simulink model "CruiseControl"  (R2024a)
settings: Solver=ode3  StartTime=0.0  StopTime=32  FixedStep=0.01  RelTol=1e-3
undefined symbols (not defined in the file): magnitude
libraries: simulink x8, SignalEditorBlockLib x1, slpidlib x1
settings Model: Creator=bnoo3  LastModifiedBy=oyj92
settings DataIOCC: SaveFormat=Array
settings ModelReferenceCC: EnableRefExpFcnMdlSchedulingChecks=on

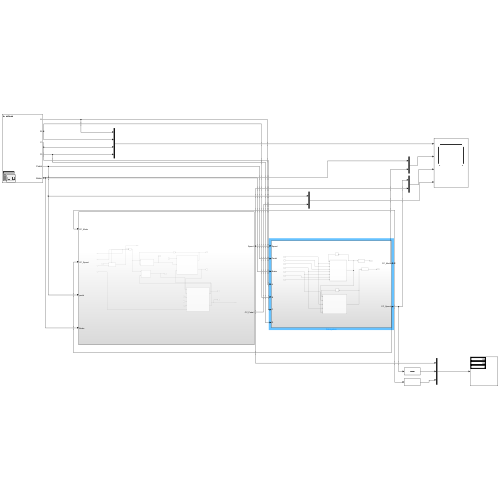
[thumbnail: Simulink's stored preview of the top-level diagram]
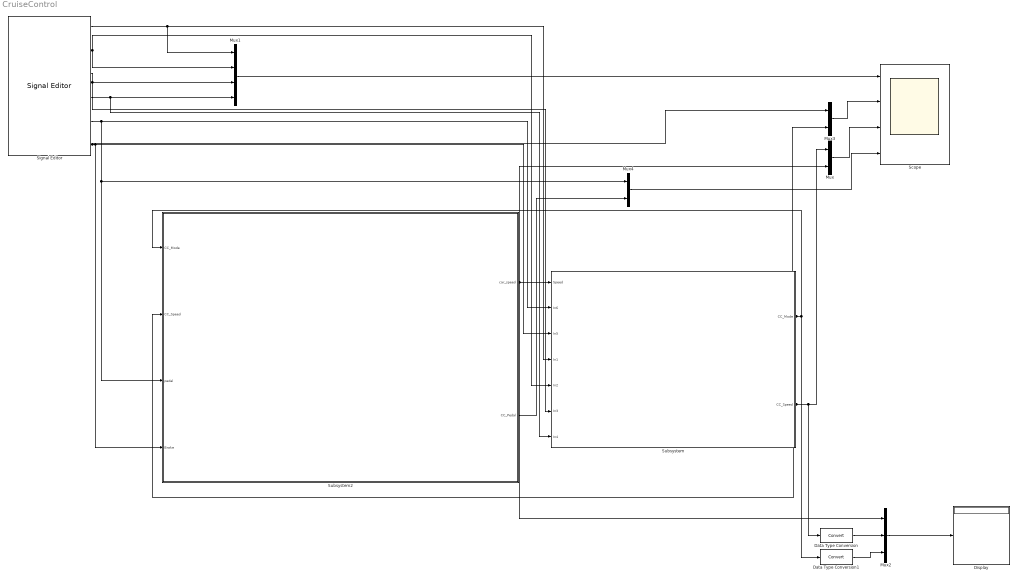
== system CruiseControl ==
  Data Type Conversion : DataTypeConversion  SaturateOnIntegerOverflow=off  RndMeth=Floor
  Data Type Conversion1 : DataTypeConversion  SaturateOnIntegerOverflow=off  RndMeth=Floor
  Display : Display
  Mux : Mux  Inputs=2
  Mux1 : Mux
  Mux2 : Mux  Inputs=3
  Mux3 : Mux  Inputs=2
  Mux4 : Mux  Inputs=2
  Scope : Scope  NumInputPorts=4
  Signal Editor : SignalEditorBlockLib/Signal Editor  FileName=C:\Users\oyj92\OneDrive\바탕 화면\OneDrive\대학교\2024-2\전장시\Ch8_CruiseControl\ref\Scenario_Result\Scenario2.mat  ActiveScenario=Scenario2  ActiveSignal=Brake  IsBus=off  OutputBusObjectStr=Bus: BusObject  SampleTime=0  Interpolate=off  ZeroCross=off  OutputAfterFinalValue=Setting to zero  Unit=inherit  PreserveSignalName=on  ApplySigPropsToAllScenarios=on  ApplySigPropsToAllSignals=off
  Subsystem : Subsystem
  Subsystem2 : Subsystem
  wires:
  Signal Editor/2 -> Mux1/2, Subsystem/5(In2)
  Signal Editor/4 -> Subsystem/7(In4), Mux1/4
  Signal Editor/6 -> Subsystem2/4(Brake), Subsystem/3(In5), Mux3/1
  Signal Editor/1 -> Subsystem/4(In1), Mux1/1
  Signal Editor/3 -> Mux1/3, Subsystem/6(In3)
  Signal Editor/5 -> Subsystem2/3(pedal), Mux4/1, Subsystem/2(In6)
  Mux/1 -> Scope/3
  Mux1/1 -> Scope/1
  Subsystem2/1(car_speed) -> Mux/2, Mux2/1, Subsystem/1(Speed)
  Subsystem2/2(CC_Pedal) -> Mux4/2
  Mux4/1 -> Scope/4
  Subsystem/1(CC_Mode) -> Mux3/2, Subsystem2/1(CC_Mode), Data Type Conversion1/1
  Subsystem/2(CC_Speed) -> Subsystem2/2(CC_Speed), Mux/1, Data Type Conversion/1
  Mux3/1 -> Scope/2
  Data Type Conversion1/1 -> Mux2/3
  Data Type Conversion/1 -> Mux2/2
  Mux2/1 -> Display/1

== system CruiseControl/Subsystem ==
  Speed : Inport
  In6 : Inport  Port=2
  In5 : Inport  Port=3
  In1 : Inport  Port=4
  In2 : Inport  Port=5
  In3 : Inport  Port=6
  In4 : Inport  Port=7
  CC ON/OFF : Subsystem
  CC SPEED Calculator : Subsystem
  Data Type Conversion : DataTypeConversion  SaturateOnIntegerOverflow=off  RndMeth=Floor
  Data Type Conversion1 : DataTypeConversion  SaturateOnIntegerOverflow=off  RndMeth=Floor
  Unit Delay : UnitDelay  SampleTime=0.01  HasFrameUpgradeWarning=on
  Unit Delay1 : UnitDelay  SampleTime=0.01  HasFrameUpgradeWarning=on
  CC_Mode : Outport
  CC_Speed : Outport  Port=2  OutMin=0  OutMax=255  OutDataTypeStr=int16
  wires:
  CC ON/OFF/1(CC_Mode) -> CC SPEED Calculator/2(Speed), Unit Delay/1, Data Type Conversion/1
  In1/1 -> CC SPEED Calculator/4(A), CC ON/OFF/5(In3)  "A"
  In2/1 -> CC SPEED Calculator/5(B), CC ON/OFF/6(In4)  "B"
  In3/1 -> CC ON/OFF/7(In5)  "C"
  In5/1 -> CC ON/OFF/4(Brake)  "Brake"
  Unit Delay/1 -> CC ON/OFF/1(In1)
  In4/1 -> CC ON/OFF/8(In6)  "D"
  Speed/1 -> CC SPEED Calculator/3(In2), CC ON/OFF/2(Speed)  "Speed"
  In6/1 -> CC ON/OFF/3(Pedal)  "Pedal"
  CC SPEED Calculator/1(CC_speed) -> Unit Delay1/1, Data Type Conversion1/1
  Unit Delay1/1 -> CC SPEED Calculator/1(In1)
  Data Type Conversion/1 -> CC_Mode/1  "CC_Mode"
  Data Type Conversion1/1 -> CC_Speed/1  "CC_Speed"

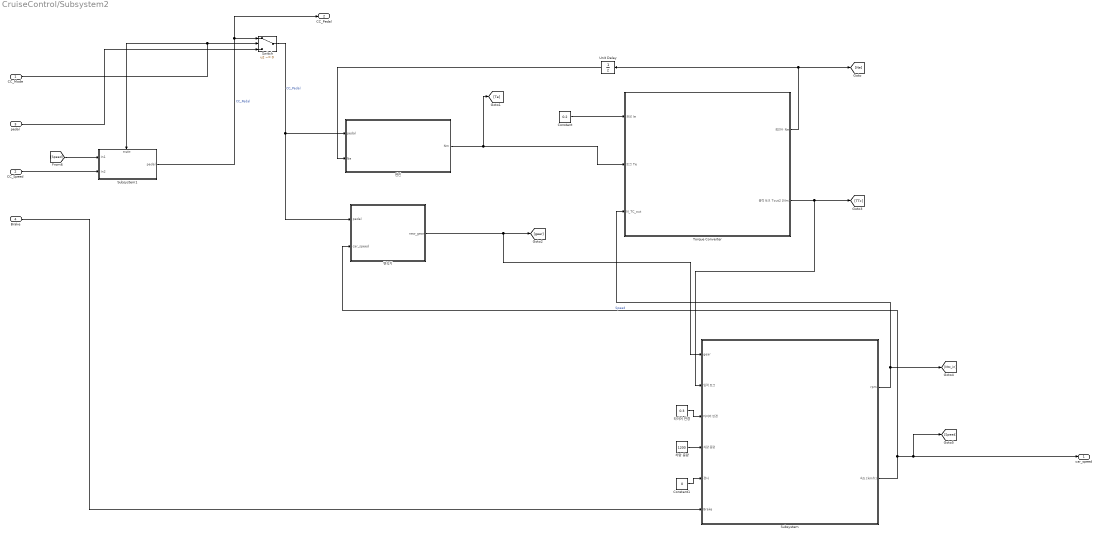
== system CruiseControl/Subsystem2 ==
  CC_Mode : Inport
  CC_Speed : Inport  Port=2
  pedal : Inport  Port=3
  Brake : Inport  Port=4
  Constant : Constant  Value=0.2
  Constant1 : Constant  Value=0
  Subsystem : Subsystem
  Subsystem1 : Subsystem
  Switch : Switch  Criteria=u2 ~= 0  SaturateOnIntegerOverflow=off  InputSameDT=off
  Torque Converter : Subsystem
  Unit Delay : UnitDelay  SampleTime=-1  HasFrameUpgradeWarning=on
  변속기 : Subsystem
  엔진 : Subsystem
  차량 중량 : Constant  Value=1200
  타이어 반경 : Constant  Value=0.3
  car_speed : Outport
  CC_Pedal : Outport  Port=2
  wires:
  Switch/1 -> 엔진/1(pedal), 변속기/1(pedal)  "CC_Pedal"
  CC_Mode/1 -> Subsystem1/Enable, Switch/2
  Unit Delay/1 -> 엔진/2(Ne)
  Subsystem/2(속도 [km/h]) -> 변속기/2(car_speed), car_speed/1, [Speed]  "Speed"
  타이어 반경/1 -> Subsystem/3(타이어 반경)
  CC_Speed/1 -> Subsystem1/2(In2)
  엔진/1(Nm) -> [Te], Torque Converter/2(토크 Te)
  pedal/1 -> Switch/3
  변속기/1(new_gear) -> [gear], Subsystem/1(gear)
  Constant1/1 -> Subsystem/5(경사)
  Torque Converter/2(출력 토크 Tout2 [Nm]) -> [TTc], Subsystem/2(입력 토크)
  Subsystem1/1(pedal) -> CC_Pedal/1, Switch/1  "CC_Pedal"
  Brake/1 -> Subsystem/6(Brake)
  Constant/1 -> Torque Converter/1(관성 Ie)
  Subsystem/1(rpm) -> Torque Converter/3(N_TC_out), [Ntc_in]
  Torque Converter/1(회전수 Ne) -> Unit Delay/1, [Ne]
  [Speed] -> Subsystem1/1(In1)
  차량 중량/1 -> Subsystem/4(차량 중량)

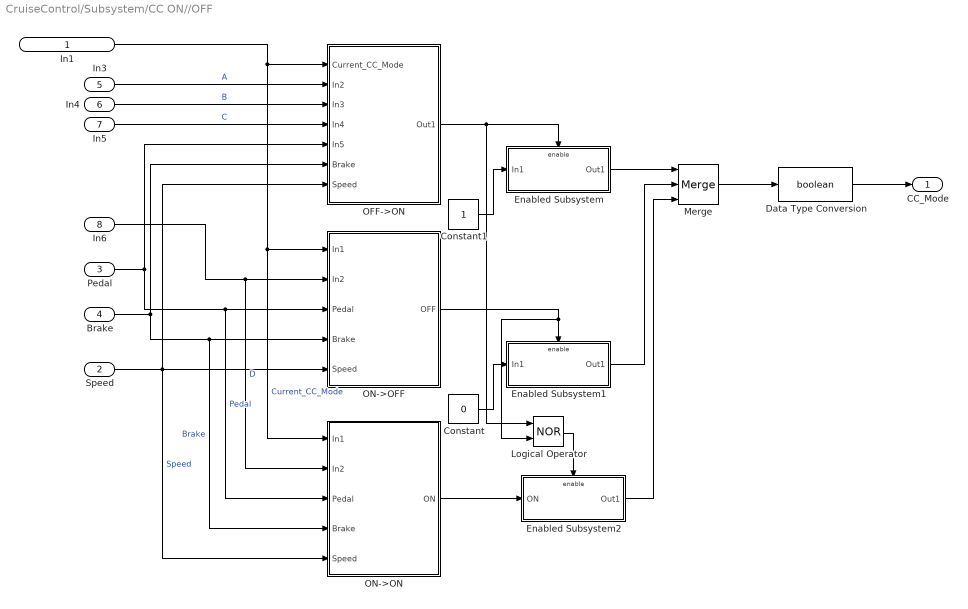
== system CruiseControl/Subsystem/CC ON//OFF ==
  In1 : Inport
  Speed : Inport  Port=2
  Pedal : Inport  Port=3
  Brake : Inport  Port=4
  In3 : Inport  Port=5
  In4 : Inport  Port=6
  In5 : Inport  Port=7
  In6 : Inport  Port=8
  Constant : Constant  Value=0
  Constant1 : Constant
  Data Type Conversion : DataTypeConversion  OutDataTypeStr=boolean  SaturateOnIntegerOverflow=off  RndMeth=Floor
  Enabled Subsystem : Subsystem  TreatAsAtomicUnit=on
  Enabled Subsystem1 : Subsystem  TreatAsAtomicUnit=on
  Enabled Subsystem2 : Subsystem  TreatAsAtomicUnit=on
  Logical Operator : Logic  Operator=NOR  AllPortsSameDT=off  OutDataTypeStr=boolean
  Merge : Merge  Inputs=3
  OFF->ON : Subsystem
  ON->OFF : Subsystem
  ON->ON : Subsystem
  CC_Mode : Outport
  wires:
  Data Type Conversion/1 -> CC_Mode/1
  ON->ON/1(ON) -> Enabled Subsystem2/1(ON)
  Enabled Subsystem2/1(Out1) -> Merge/3
  Speed/1 -> OFF->ON/7(Speed), ON->ON/5(Speed), ON->OFF/5(Speed)  "Speed"
  Enabled Subsystem/1(Out1) -> Merge/1
  In1/1 -> ON->ON/1(In1), ON->OFF/1(In1), OFF->ON/1(Current_CC_Mode)  "Current_CC_Mode"
  Enabled Subsystem1/1(Out1) -> Merge/2
  Merge/1 -> Data Type Conversion/1
  In5/1 -> OFF->ON/4(In4)  "C"
  In3/1 -> OFF->ON/2(In2)  "A"
  OFF->ON/1(Out1) -> Enabled Subsystem/Enable, Logical Operator/1
  Pedal/1 -> ON->ON/3(Pedal), ON->OFF/3(Pedal), OFF->ON/5(In5)  "Pedal"
  In6/1 -> ON->ON/2(In2), ON->OFF/2(In2)  "D"
  ON->OFF/1(OFF) -> Logical Operator/2, Enabled Subsystem1/Enable
  Constant/1 -> Enabled Subsystem1/1(In1)
  Brake/1 -> ON->ON/4(Brake), ON->OFF/4(Brake), OFF->ON/6(Brake)  "Brake"
  Constant1/1 -> Enabled Subsystem/1(In1)
  In4/1 -> OFF->ON/3(In3)  "B"
  Logical Operator/1 -> Enabled Subsystem2/Enable

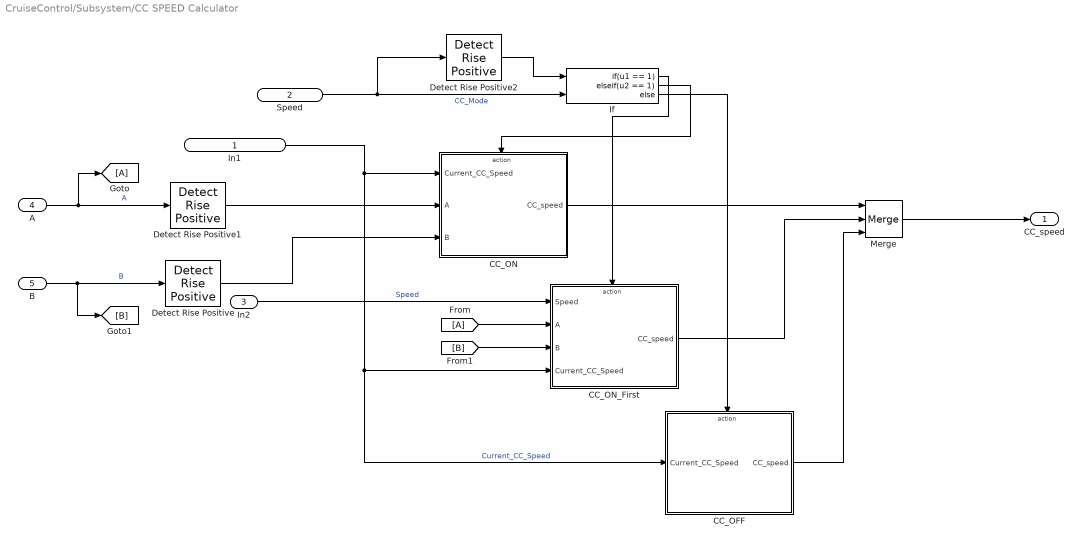
== system CruiseControl/Subsystem/CC SPEED Calculator ==
  In1 : Inport
  Speed : Inport  Port=2
  In2 : Inport  Port=3
  A : Inport  Port=4
  B : Inport  Port=5
  CC_OFF : Subsystem  TreatAsAtomicUnit=on
  CC_ON : Subsystem  TreatAsAtomicUnit=on
  CC_ON_First : Subsystem  TreatAsAtomicUnit=on
  Detect Rise Positive : simulink/Logic and Bit Operations/Detect Rise Positive  vinit=0  OutDataTypeStr=boolean
  Detect Rise Positive1 : simulink/Logic and Bit Operations/Detect Rise Positive  vinit=0  OutDataTypeStr=boolean
  Detect Rise Positive2 : simulink/Logic and Bit Operations/Detect Rise Positive  vinit=0  OutDataTypeStr=boolean
  From : From
  Goto : Goto
  If : If  NumInputs=2  IfExpression=u1 == 1  ElseIfExpressions=u2 == 1
  Merge : Merge  Inputs=3
  CC_speed : Outport
  wires:
  A/1 -> Goto/1, Detect Rise Positive1/1  "A"
  From/1 -> CC_ON_First/2(A)
  Detect Rise Positive/1 -> CC_ON/3(B)
  Speed/1 -> Detect Rise Positive2/1, If/2  "CC_Mode"
  [B] -> CC_ON_First/3(B)
  B/1 -> [B], Detect Rise Positive/1  "B"
  If/2 -> CC_ON/Action
  Detect Rise Positive1/1 -> CC_ON/2(A)
  Merge/1 -> CC_speed/1
  If/1 -> CC_ON_First/Action
  In1/1 -> CC_OFF/1(Current_CC_Speed), CC_ON_First/4(Current_CC_Speed), CC_ON/1(Current_CC_Speed)  "Current_CC_Speed"
  If/3 -> CC_OFF/Action
  In2/1 -> CC_ON_First/1(Speed)  "Speed"
  CC_OFF/1(CC_speed) -> Merge/3
  CC_ON/1(CC_speed) -> Merge/1
  CC_ON_First/1(CC_speed) -> Merge/2
  Detect Rise Positive2/1 -> If/1

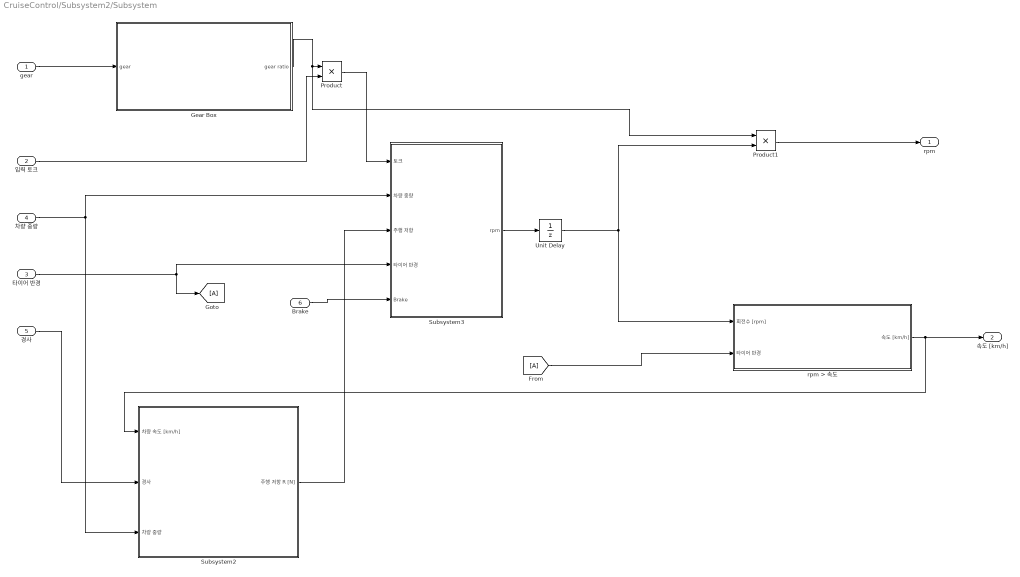
== system CruiseControl/Subsystem2/Subsystem ==
  gear : Inport
  입력 토크 : Inport  Port=2
  타이어 반경 : Inport  Port=3
  차량 중량 : Inport  Port=4
  경사 : Inport  Port=5
  Brake : Inport  Port=6
  From : From
  Gear Box : Subsystem
  Goto : Goto
  Product : Product
  Product1 : Product
  Subsystem2 : Subsystem
  Subsystem3 : Subsystem
  Unit Delay : UnitDelay  SampleTime=-1  HasFrameUpgradeWarning=on
  rpm > 속도 : Subsystem
  rpm : Outport
  속도 [km/h] : Outport  Port=2
  wires:
  경사/1 -> Subsystem2/2(경사)
  rpm > 속도/1(속도 [km/h]) -> 속도 [km/h]/1, Subsystem2/1(차량 속도 [km/h])
  From/1 -> rpm > 속도/2(타이어 반경)
  Subsystem3/1(rpm) -> Unit Delay/1
  차량 중량/1 -> Subsystem2/3(차량 중량), Subsystem3/2(차량 중량)
  Subsystem2/1(주행 저항 R [N]) -> Subsystem3/3(주행 저항)
  입력 토크/1 -> Product/2
  타이어 반경/1 -> Goto/1, Subsystem3/4(타이어 반경)
  gear/1 -> Gear Box/1(gear)
  Gear Box/1(gear ratio) -> Product1/1, Product/1
  Product/1 -> Subsystem3/1(토크)
  Product1/1 -> rpm/1
  Unit Delay/1 -> Product1/2, rpm > 속도/1(회전수 [rpm])
  Brake/1 -> Subsystem3/5(Brake)

== system CruiseControl/Subsystem2/Subsystem1 ==
  In1 : Inport
  In2 : Inport  Port=2
  Enable : EnablePort  StatesWhenEnabling=reset
  Data Type Conversion1 : DataTypeConversion  SaturateOnIntegerOverflow=off  RndMeth=Floor
  Discrete PID Controller : slpidlib/PID Controller  Controller=PID  Form=Parallel  TimeDomain=Discrete-time  UseExternalTs=off  SampleTime=0.01  IntegratorMethod=Forward Euler  FilterMethod=Forward Euler  ControllerParametersSource=internal  P=2  I=4  UseKiTs=off  D=0  UseExternalDerivativeSource=off  N=100  UseFilter=on  TunerSelectOption=Transfer Function Based (PID Tuner App)  InitialConditionSource=internal  InitialConditionForIntegrator=0  InitialConditionForFilter=0  DifferentiatorICPrevScaledInput=0  ExternalReset=none  TrackingMode=off  Kt=1  LimitOutput=on  SatLimitsSource=internal  UpperSaturationLimit=80  LowerSaturationLimit=0  LinearizeAsGain=off  AntiWindupMode=none  Kb=1  LimitIntegrator=off  UpperIntegratorSaturationLimit=inf  LowerIntegratorSaturationLimit=-inf  POutMin=[]  POutMax=[]  IOutMin=[]  IOutMax=[]  DOutMin=[]  DOutMax=[]  NOutMin=[]  NOutMax=[]  SumOutMin=[]  SumOutMax=[]  SaturationOutMin=[]  SaturationOutMax=[]  PParamMin=[]  PParamMax=[]  IParamMin=[]  IParamMax=[]  DParamMin=[]  DParamMax=[]  NParamMin=[]  NParamMax=[]  KbParamMin=[]  KbParamMax=[]  KtParamMin=[]  KtParamMax=[]  KbOutMin=[]  KbOutMax=[]  KtOutMin=[]  KtOutMax=[]  IntegratorOutMin=[]  IntegratorOutMax=[]  FilterOutMin=[]  FilterOutMax=[]  SumI1OutMin=[]  SumI1OutMax=[]  SumI2OutMin=[]  SumI2OutMax=[]  SumI3OutMin=[]  SumI3OutMax=[]  SumI4OutMin=[]  SumI4OutMax=[]  SumDOutMin=[]  SumDOutMax=[]  DifferentiatorOutMin=[]  DifferentiatorOutMax=[]  FilterDiffOutCoefMin=[]  FilterDiffOutCoefMax=[]  ReciprocalOutMin=[]  ReciprocalOutMax=[]  SumDenOutMin=[]  SumDenOutMax=[]  SumNumOutMin=[]  SumNumOutMax=[]  DivideOutMin=[]  DivideOutMax=[]  UdiffTsProdOutMin=[]  UdiffTsProdOutMax=[]  NTsProdOutMin=[]  NTsProdOutMax=[]  UintegralTsProdOutMin=[]  UintegralTsProdOutMax=[]  UngainTsProdOutMin=[]  UngainTsProdOutMax=[]  ClampingZeroOutDataTypeStr=Inherit: Inherit via back propagation  ClampingZeroOutMin=[]  ClampingZeroOutMax=[]  FilterDenConstantOutDataTypeStr=Inherit: Inherit via back propagation  FilterDenConstantOutMin=[]  FilterDenConstantOutMax=[]  PCopyOutDataTypeStr=Inherit: Inherit via back propagation  PCopyOutMin=[]  PCopyOutMax=[]  NCopyOutDataTypeStr=Inherit: Inherit via back propagation  NCopyOutMin=[]  NCopyOutMax=[]  IntegratorContinuousStateAttributes=''  IntegratorStateMustResolveToSignalObject=off  IntegratorRTWStateStorageClass=Auto  FilterContinuousStateAttributes=''  FilterStateMustResolveToSignalObject=off  FilterRTWStateStorageClass=Auto  ParallelPVariant=InternalParameters  IdealPVariant=Disabled  IVariant=InternalParameters  DVariant=InternalParameters  IntegratorVariant=Discrete  SatVariant=Enabled  AWVariant=Passthrough  PCopyVariant=Disabled  TRVariant=Disabled  FdbkBlocksVariant=Forward  IdealPFdbkVariant=Disabled  SatFdbkVariant=Disabled  DerivativeFilterVariant=ForwardEulerFilter  NVariant=InternalParameters  NCopyVariant=Disabled  FilterICVariant=InternalICsFilter  IntegratorICVariant=InternalICs  ExternalResetVariant=Disabled  TRSumVariant=Passthrough  SumFdbkVariant=Disabled  SumVariant=Sum_PID  TsampFilterVariant=InternalTs  TsampNgainVariant=Passthrough  TsampIntegralVariant=Disabled_SignalSpec  ExternalSaturationOutDataTypeStr=Inherit: Same as second input  DerivativeSourceVariant=ErrorSignal
      settings: LibrarySourceBlock=simulink/Discrete/Discrete PID Controller
  Saturation : Saturate  UpperLimit=10  LowerLimit=-10
  Subtract : Sum  Inputs=+-
  pedal : Outport
  wires:
  In1/1 -> Subtract/2
  Subtract/1 -> Saturation/1
  Saturation/1 -> Data Type Conversion1/1
  In2/1 -> Subtract/1
  Discrete PID Controller/1 -> pedal/1
  Data Type Conversion1/1 -> Discrete PID Controller/1

== system CruiseControl/Subsystem2/Torque Converter ==
  관성 Ie : Inport
  토크 Te : Inport  Port=2
  N_TC_out : Inport  Port=3
  Scope : Scope  NumInputPorts=2
  Scope1 : Scope  NumInputPorts=2
  Subtract : Sum  Inputs=+-
  Unit Delay : UnitDelay  SampleTime=-1  HasFrameUpgradeWarning=on
  각가속도 > 각속도 : Subsystem
  각속도 > rpm : Subsystem
  토크 > 각가속도 : Subsystem
  회전수 > 토크 : Subsystem
  회전수 Ne : Outport
  출력 토크 Tout2 [Nm] : Outport  Port=2
  wires:
  관성 Ie/1 -> 토크 > 각가속도/1(I [kgm^2])
  토크 > 각가속도/1(W) -> 각가속도 > 각속도/1(각가속도 [rad/sec^2])
  각가속도 > 각속도/1(각속도 [rad/sec]) -> 각속도 > rpm/1(rad/sec)
  각속도 > rpm/1(rpm) -> Scope/1, 회전수 > 토크/1(엔진 회전수 Ne [rpm]), 회전수 Ne/1
  회전수 > 토크/2(출력 토크 Tout2 [Nm]) -> 출력 토크 Tout2 [Nm]/1, Scope/2
  N_TC_out/1 -> 회전수 > 토크/2(출력 회전수 Nout [rpm])
  Subtract/1 -> 토크 > 각가속도/2(T [Nm])
  토크 Te/1 -> Subtract/1
  회전수 > 토크/1(균형 토크 Tout1 [Nm]) -> Unit Delay/1, Scope1/1
  회전수 > 토크/3(속도비 e) -> Scope1/2
  Unit Delay/1 -> Subtract/2

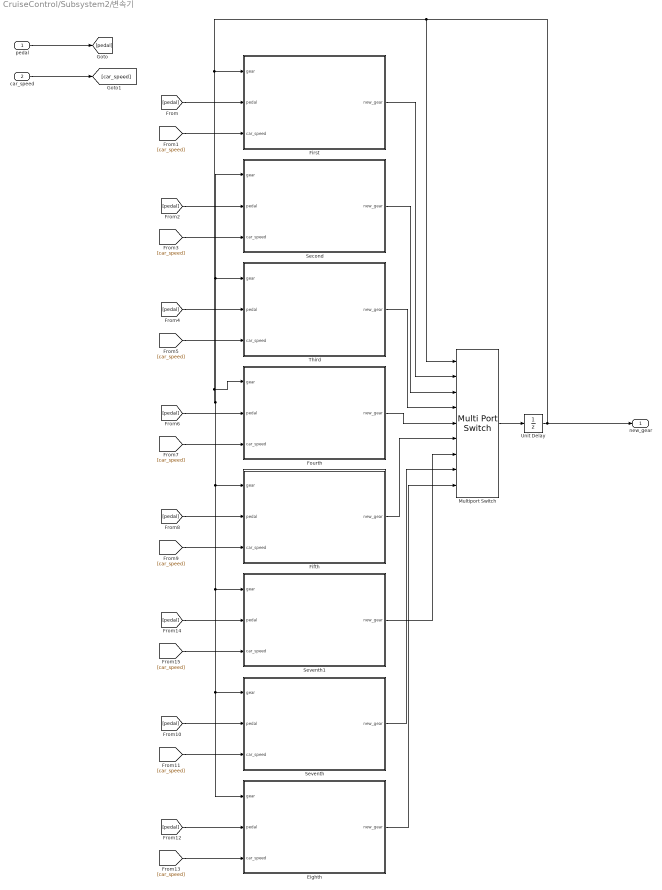
== system CruiseControl/Subsystem2/변속기 ==
  pedal : Inport
  car_speed : Inport  Port=2
  Eighth : Subsystem
  Fifth : Subsystem
  First : Subsystem
  Fourth : Subsystem
  Multiport Switch : MultiPortSwitch  Inputs=8  OutMin=[60]  SaturateOnIntegerOverflow=off  InputSameDT=off
  Second : Subsystem
  Seventh : Subsystem
  Seventh1 : Subsystem
  Third : Subsystem
  Unit Delay : UnitDelay  InitialCondition=1  SampleTime=-1  HasFrameUpgradeWarning=on
  new_gear : Outport
  wires:
  Seventh/1(new_gear) -> Multiport Switch/8
  [car_speed] -> Eighth/3(car_speed)
  Fourth/1(new_gear) -> Multiport Switch/5
  Eighth/1(new_gear) -> Multiport Switch/9
  [car_speed] -> Seventh/3(car_speed)
  First/1(new_gear) -> Multiport Switch/2
  [pedal] -> Third/2(pedal)
  [car_speed] -> Fourth/3(car_speed)
  [pedal] -> Eighth/2(pedal)
  [pedal] -> Fifth/2(pedal)
  Third/1(new_gear) -> Multiport Switch/4
  [pedal] -> Fourth/2(pedal)
  pedal/1 -> [pedal]
  [car_speed] -> Fifth/3(car_speed)
  [pedal] -> Second/2(pedal)
  [car_speed] -> Third/3(car_speed)
  car_speed/1 -> [car_speed]
  Fifth/1(new_gear) -> Multiport Switch/6
  [pedal] -> Seventh/2(pedal)
  [pedal] -> First/2(pedal)
  [car_speed] -> First/3(car_speed)
  [car_speed] -> Second/3(car_speed)
  Second/1(new_gear) -> Multiport Switch/3
  Multiport Switch/1 -> Unit Delay/1
  [pedal] -> Seventh1/2(pedal)
  [car_speed] -> Seventh1/3(car_speed)
  Unit Delay/1 -> Multiport Switch/1, Fourth/1(gear), Eighth/1(gear), Seventh/1(gear), Seventh1/1(gear), Fifth/1(gear), Third/1(gear), Second/1(gear), First/1(gear), new_gear/1
  Seventh1/1(new_gear) -> Multiport Switch/7

== system CruiseControl/Subsystem2/엔진 ==
  pedal : Inport
  Ne : Inport  Port=2
  Nm Calculate : Lookup_n-D  BreakpointsForDimension1=[0 2 5 10 15 20 25 30 35 40 50 60 70 80 90 100]  BreakpointsForDimension2=[-10, 450, 500, 750, 1000, 1250, 1500, 1750, 2000, 2500, 3000, 3500, 4000, 4500, 5000, 5500, 6000, 6300, 6500]  Table=[0, 0, 7, 16, 28, 10, -17, -20, -22, -25, -28, -31, -34, -39, -43, -49, -54, -54, -54; 0, 0, 17, 29, 46, 15, 0, -6, -11, -22, -28, -31, -34, -39, -43, -49, -54, -54, -54; 0, 0, 31, 38, 51, 23, 15, 8, 3, -10, -17, -22, -26, -30, -34, -38, -43, -43, -43; 0, 0, 55, 46, 41, 36, 31, 27, 23, 16, 10, 3, -5, -8, -10, -13, -15, -15, -15; 0, 0, 60, 56, 54, 51, 48, 44, 40, 32, 25, 19, 13, 10, 7, 5, 3, 3, 3; 0, 0, 65, 66, 66, 66, 64, 61, 57, 48, 40, 35, 30, 27, 24, 20, 20, 20, 20; 0, 0, 70, 75, 78, 81, 81, 79, 75, 65, 55, 49, 43, 38, 34, 31, 29, 29, 29; 0, 0, 75, 83, 90, 96, 98, 97, 93, 80, 70, 63, 55, 50, 44, 41, 37, 37, 37; 0, 0, 79, 90, 100, 109, 114, 115, 112, 96, 85, 77, 68, 63, 58, 55, 51, 51, 51; 0, 0, 82, 96, 109, 121, 129, 132, 130, 112, 100, 91, 81, 77, 72, 69, 65, 65, 65; 0, 0, 103, 114, 130, 148, 164, 171, 170, 156, 140, 128, 116, 111, 105, 100, 95, 95, 95; 0, 0, 148, 155, 168, 189, 210, 224, 224, 210, 183, 167, 150, 142, 133, 128, 123, 123, 123; 0, 0, 150, 160, 170, 190, 210, 230, 260, 255, 225, 203, 180, 168, 156, 151, 145, 145, 145; 0, 0, 150, 160, 170, 190, 210, 230, 260, 290, 260, 233, 206, 191, 176, 173, 170, 170, 170; 0, 0, 150, 160, 170, 190, 210, 230, 260, 320, 300, 276, 252, 233, 213, 209, 204, 204, 204; 0, 0, 150, 160, 170, 190, 210, 230, 260, 330, 319, 302, 285, 266, 246, 243, 239, 239, 239]  InternalRulePriority=Speed  RndMeth=Simplest
      settings: InputPortMap=u0,u1
  Step : Step  Before=100  After=0  SampleTime=0
  Switch : Switch  Criteria=u2 ~= 0  SaturateOnIntegerOverflow=off  InputSameDT=off
  Nm : Outport
  wires:
  Nm Calculate/1 -> Switch/3
  Step/1 -> Switch/2, Switch/1
  pedal/1 -> Nm Calculate/1
  Ne/1 -> Nm Calculate/2
  Switch/1 -> Nm/1

== system CruiseControl/Subsystem/CC ON//OFF/Enabled Subsystem ==
  In1 : Inport
  Enable : EnablePort
  Out1 : Outport
  wires:
  In1/1 -> Out1/1

== system CruiseControl/Subsystem/CC ON//OFF/Enabled Subsystem1 ==
  In1 : Inport
  Enable : EnablePort
  Out1 : Outport
  wires:
  In1/1 -> Out1/1

== system CruiseControl/Subsystem/CC ON//OFF/Enabled Subsystem2 ==
  ON : Inport
  Enable : EnablePort
  Out1 : Outport
  wires:
  ON/1 -> Out1/1

== system CruiseControl/Subsystem/CC ON//OFF/OFF->ON ==
  Current_CC_Mode : Inport
  In2 : Inport  Port=2
  In3 : Inport  Port=3
  In4 : Inport  Port=4
  In5 : Inport  Port=5
  Brake : Inport  Port=6
  Speed : Inport  Port=7
  Constant : Constant  Value=65
  Interval Test : simulink/Logic and Bit Operations/Interval Test  IntervalClosedRight=on  uplimit=110  IntervalClosedLeft=on  lowlimit=55  OutDataTypeStr=boolean
  Logical Operator : Logic  Operator=OR  Inputs=3  AllPortsSameDT=off  OutDataTypeStr=boolean
  Logical Operator1 : Logic  Inputs=5  AllPortsSameDT=off  OutDataTypeStr=boolean
  Logical Operator2 : Logic  Operator=NOT  AllPortsSameDT=off  OutDataTypeStr=boolean
  Logical Operator3 : Logic  Operator=NOT  AllPortsSameDT=off  OutDataTypeStr=boolean
  Relational Operator : RelationalOperator  Operator=<  OutDataTypeStr=boolean  RndMeth=Simplest  InputSameDT=off
  Out1 : Outport
  wires:
  In2/1 -> Logical Operator/1  "A"
  In3/1 -> Logical Operator/2  "B"
  In4/1 -> Logical Operator/3  "C"
  In5/1 -> Relational Operator/1  "Pedal"
  Constant/1 -> Relational Operator/2
  Speed/1 -> Interval Test/1  "Speed"
  Logical Operator/1 -> Logical Operator1/2
  Relational Operator/1 -> Logical Operator1/3
  Interval Test/1 -> Logical Operator1/5
  Logical Operator1/1 -> Out1/1  "ON"
  Brake/1 -> Logical Operator2/1  "Brake"
  Logical Operator2/1 -> Logical Operator1/4
  Current_CC_Mode/1 -> Logical Operator3/1
  Logical Operator3/1 -> Logical Operator1/1

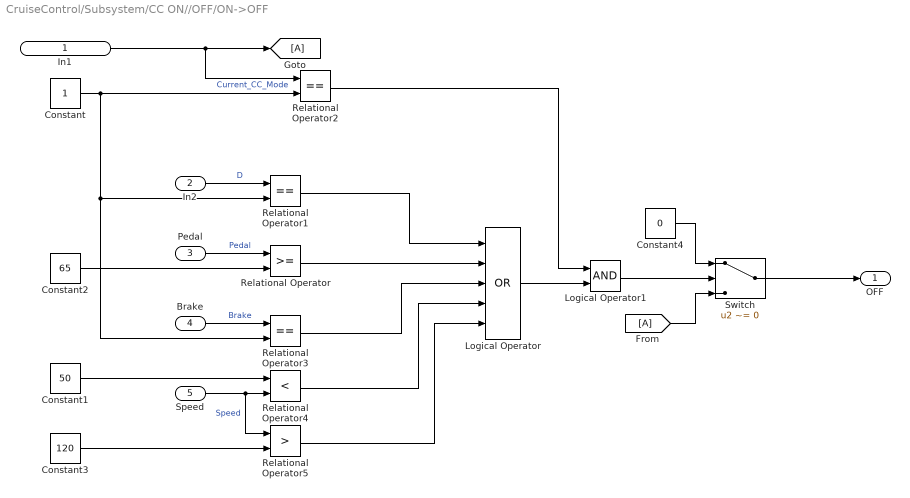
== system CruiseControl/Subsystem/CC ON//OFF/ON->OFF ==
  In1 : Inport
  In2 : Inport  Port=2
  Pedal : Inport  Port=3
  Brake : Inport  Port=4
  Speed : Inport  Port=5
  Constant : Constant
  Constant1 : Constant  Value=50
  Constant2 : Constant  Value=65
  Constant3 : Constant  Value=120
  Constant4 : Constant  Value=0
  From : From
  Goto : Goto
  Logical Operator : Logic  Operator=OR  Inputs=5  AllPortsSameDT=off  OutDataTypeStr=boolean
  Logical Operator1 : Logic  AllPortsSameDT=off  OutDataTypeStr=boolean
  Relational Operator : RelationalOperator  OutDataTypeStr=boolean  RndMeth=Simplest  InputSameDT=off
  Relational Operator1 : RelationalOperator  Operator===  OutDataTypeStr=boolean  RndMeth=Simplest  InputSameDT=off
  Relational Operator2 : RelationalOperator  Operator===  OutDataTypeStr=boolean  RndMeth=Simplest  InputSameDT=off
  Relational Operator3 : RelationalOperator  Operator===  OutDataTypeStr=boolean  RndMeth=Simplest  InputSameDT=off
  Relational Operator4 : RelationalOperator  Operator=<  OutDataTypeStr=boolean  RndMeth=Simplest  InputSameDT=off
  Relational Operator5 : RelationalOperator  Operator=>  OutDataTypeStr=boolean  RndMeth=Simplest  InputSameDT=off
  Switch : Switch  Criteria=u2 ~= 0  SaturateOnIntegerOverflow=off  InputSameDT=off
  OFF : Outport
  wires:
  In1/1 -> Relational Operator2/1, Goto/1  "Current_CC_Mode"
  Constant/1 -> Relational Operator3/2, Relational Operator1/2, Relational Operator2/2
  In2/1 -> Relational Operator1/1  "D"
  Relational Operator1/1 -> Logical Operator/1
  Pedal/1 -> Relational Operator/1  "Pedal"
  Constant2/1 -> Relational Operator/2
  Relational Operator/1 -> Logical Operator/2
  Brake/1 -> Relational Operator3/1  "Brake"
  Speed/1 -> Relational Operator5/1, Relational Operator4/2  "Speed"
  Constant3/1 -> Relational Operator5/2
  Constant1/1 -> Relational Operator4/1
  Relational Operator3/1 -> Logical Operator/3
  Relational Operator4/1 -> Logical Operator/4
  Relational Operator5/1 -> Logical Operator/5
  Relational Operator2/1 -> Logical Operator1/1
  Logical Operator/1 -> Logical Operator1/2
  Logical Operator1/1 -> Switch/2
  Constant4/1 -> Switch/1
  From/1 -> Switch/3
  Switch/1 -> OFF/1

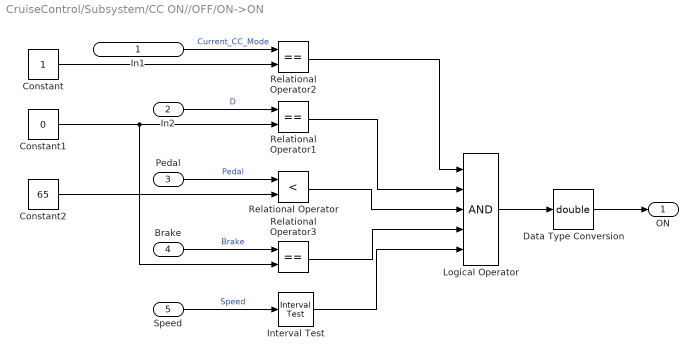
== system CruiseControl/Subsystem/CC ON//OFF/ON->ON ==
  In1 : Inport
  In2 : Inport  Port=2
  Pedal : Inport  Port=3
  Brake : Inport  Port=4
  Speed : Inport  Port=5
  Constant : Constant
  Constant1 : Constant  Value=0
  Constant2 : Constant  Value=65
  Data Type Conversion : DataTypeConversion  OutDataTypeStr=double  RndMeth=Nearest  SaturateOnIntegerOverflow=off
  Interval Test : simulink/Logic and Bit Operations/Interval Test  IntervalClosedRight=on  uplimit=120  IntervalClosedLeft=on  lowlimit=50  OutDataTypeStr=boolean
  Logical Operator : Logic  Inputs=5  AllPortsSameDT=off  OutDataTypeStr=boolean
  Relational Operator : RelationalOperator  Operator=<  OutDataTypeStr=boolean  RndMeth=Simplest  InputSameDT=off
  Relational Operator1 : RelationalOperator  Operator===  OutDataTypeStr=boolean  RndMeth=Simplest  InputSameDT=off
  Relational Operator2 : RelationalOperator  Operator===  OutDataTypeStr=boolean  RndMeth=Simplest  InputSameDT=off
  Relational Operator3 : RelationalOperator  Operator===  OutDataTypeStr=boolean  RndMeth=Simplest  InputSameDT=off
  ON : Outport
  wires:
  In1/1 -> Relational Operator2/1  "Current_CC_Mode"
  Constant/1 -> Relational Operator2/2
  In2/1 -> Relational Operator1/1  "D"
  Relational Operator1/1 -> Logical Operator/2
  Pedal/1 -> Relational Operator/1  "Pedal"
  Constant2/1 -> Relational Operator/2
  Relational Operator/1 -> Logical Operator/3
  Brake/1 -> Relational Operator3/1  "Brake"
  Speed/1 -> Interval Test/1  "Speed"
  Relational Operator3/1 -> Logical Operator/4
  Relational Operator2/1 -> Logical Operator/1
  Logical Operator/1 -> Data Type Conversion/1
  Constant1/1 -> Relational Operator3/2, Relational Operator1/2
  Interval Test/1 -> Logical Operator/5
  Data Type Conversion/1 -> ON/1

== system CruiseControl/Subsystem/CC SPEED Calculator/CC_OFF ==
  note: CC ON First
  Current_CC_Speed : Inport
  Action Port : ActionPort  ActionPortLabel=else
  CC_speed : Outport
  wires:
  Current_CC_Speed/1 -> CC_speed/1

== system CruiseControl/Subsystem/CC SPEED Calculator/CC_ON ==
  note: CC ON
  Current_CC_Speed : Inport
  A : Inport  Port=2
  B : Inport  Port=3
  Action Port : ActionPort  ActionPortLabel=elseif(u2 == 1)
  A 동작 : Subsystem  TreatAsAtomicUnit=on
  A,B 둘다동작X : Subsystem  TreatAsAtomicUnit=on
  B 동작 : Subsystem  TreatAsAtomicUnit=on
  Constant : Constant  SampleTime=-1
  Logical Operator : Logic  AllPortsSameDT=off  OutDataTypeStr=boolean
  Merge : Merge  Inputs=3
  NOT : Logic  Operator=NOT  IconShape=distinctive  AllPortsSameDT=off  OutDataTypeStr=boolean
  NOT1 : Logic  Operator=NOT  IconShape=distinctive  AllPortsSameDT=off  OutDataTypeStr=boolean
  Relational Operator : RelationalOperator  Operator===  OutDataTypeStr=boolean  RndMeth=Simplest  InputSameDT=off
  Relational Operator1 : RelationalOperator  Operator===  OutDataTypeStr=boolean  RndMeth=Simplest  InputSameDT=off
  CC_speed : Outport
  wires:
  B/1 -> NOT/1, Relational Operator1/1
  A/1 -> NOT1/1, Relational Operator/1
  Constant/1 -> Relational Operator1/2, Relational Operator/2
  Current_CC_Speed/1 -> A,B 둘다동작X/1(Current_CC_Speed), B 동작/1(Current_CC_Speed), A 동작/1(Current_CC_Speed)
  Merge/1 -> CC_speed/1
  Relational Operator/1 -> A 동작/Enable
  Relational Operator1/1 -> B 동작/Enable
  A 동작/1(Out1) -> Merge/1
  B 동작/1(Out1) -> Merge/2
  Logical Operator/1 -> A,B 둘다동작X/Enable
  NOT1/1 -> Logical Operator/1
  NOT/1 -> Logical Operator/2
  A,B 둘다동작X/1(Out1) -> Merge/3

== system CruiseControl/Subsystem/CC SPEED Calculator/CC_ON_First ==
  note: CC ON First
  Speed : Inport
  A : Inport  Port=2
  B : Inport  Port=3
  Current_CC_Speed : Inport  Port=4
  Action Port : ActionPort  ActionPortLabel=if(u1 == 1)
  Constant : Constant
  Logical Operator : Logic  Operator=OR  AllPortsSameDT=off  OutDataTypeStr=boolean
  Relational Operator : RelationalOperator  Operator===  OutDataTypeStr=boolean  RndMeth=Simplest  InputSameDT=off
  Relational Operator1 : RelationalOperator  Operator===  OutDataTypeStr=boolean  RndMeth=Simplest  InputSameDT=off
  Switch : Switch  Criteria=u2 ~= 0  SaturateOnIntegerOverflow=off  InputSameDT=off
  CC_speed : Outport
  wires:
  A/1 -> Relational Operator/1
  Constant/1 -> Relational Operator1/2, Relational Operator/2
  B/1 -> Relational Operator1/1
  Relational Operator/1 -> Logical Operator/1
  Relational Operator1/1 -> Logical Operator/2
  Logical Operator/1 -> Switch/2
  Speed/1 -> Switch/1
  Switch/1 -> CC_speed/1
  Current_CC_Speed/1 -> Switch/3

== system CruiseControl/Subsystem2/Subsystem/Gear Box ==
  gear : Inport
  Constant : Constant  Value=4.596
  Constant1 : Constant  Value=2.724
  Constant2 : Constant  Value=1.863
  Constant3 : Constant  Value=1.464
  Constant4 : Constant  Value=1.231
  Constant5 : Constant
  Constant6 : Constant  Value=0.824
  Constant7 : Constant  Value=0.685
  Constant8 : Constant  Value=2.937
  Multiport Switch : MultiPortSwitch  Inputs=8  SaturateOnIntegerOverflow=off  InputSameDT=off
  Product : Product
  gear ratio : Outport
  wires:
  Constant/1 -> Multiport Switch/2
  Multiport Switch/1 -> Product/1
  Constant1/1 -> Multiport Switch/3
  Constant2/1 -> Multiport Switch/4
  Constant3/1 -> Multiport Switch/5
  Constant4/1 -> Multiport Switch/6
  Constant5/1 -> Multiport Switch/7
  Constant6/1 -> Multiport Switch/8
  Constant7/1 -> Multiport Switch/9
  Constant8/1 -> Product/2
  Product/1 -> gear ratio/1
  gear/1 -> Multiport Switch/1

== system CruiseControl/Subsystem2/Subsystem/Subsystem2 ==
  차량 속도 [km/h] : Inport
  경사 : Inport  Port=2
  차량 중량 : Inport  Port=3
  Add : Sum  Inputs=+++
  Compare To Constant : simulink/Logic and Bit Operations/Compare To Constant  relop=<=  const=1  OutDataTypeStr=boolean
  Constant : Constant  Value=0
  Subsystem : Subsystem
  Subsystem1 : Subsystem
  Subsystem2 : Subsystem
  Switch : Switch  Criteria=u2 ~= 0  SaturateOnIntegerOverflow=off  InputSameDT=off
  주행 저항 R [N] : Outport
  wires:
  Subsystem2/1(도로 저항 [N]) -> Add/3
  Subsystem/1(주행저항 R [N]) -> Add/1
  Add/1 -> Switch/3
  차량 중량/1 -> Subsystem2/2(차량 중량), Subsystem1/2(차량 중량)
  차량 속도 [km/h]/1 -> Compare To Constant/1, Subsystem/1(차량 속도 [km/h])
  Subsystem1/1(경사 저항 [N]) -> Add/2
  경사/1 -> Subsystem1/1(경사), Subsystem2/1(경사)
  Constant/1 -> Switch/1
  Compare To Constant/1 -> Switch/2
  Switch/1 -> 주행 저항 R [N]/1

== system CruiseControl/Subsystem2/Subsystem/Subsystem3 ==
  토크 : Inport
  차량 중량 : Inport  Port=2
  주행 저항 : Inport  Port=3
  타이어 반경 : Inport  Port=4
  Brake : Inport  Port=5
  Scope : Scope  NumInputPorts=2
  Subsystem1 : Subsystem
  각가속도 > 각속도 : Subsystem
  각속도 > rpm : Subsystem
  관성 계산 : Subsystem
  토크 > 각가속도 : Subsystem
  rpm : Outport
  wires:
  토크 > 각가속도/1(W) -> Scope/1, 각가속도 > 각속도/1(각가속도 [rad/sec^2])
  관성 계산/1(관성) -> 토크 > 각가속도/2(I [kgm^2])
  Subsystem1/1(손실 포함 입력 토크) -> 토크 > 각가속도/1(T [Nm])
  토크/1 -> Subsystem1/1(토크)
  각가속도 > 각속도/1(각속도 [rad/sec]) -> Scope/2, 각속도 > rpm/1(rad/sec)
  주행 저항/1 -> Subsystem1/2(주행 저항)
  타이어 반경/1 -> Subsystem1/3(타이어 반경), 관성 계산/2(타이어 반경)
  차량 중량/1 -> 관성 계산/1(차량 중량)
  각속도 > rpm/1(rpm) -> rpm/1
  Brake/1 -> Subsystem1/4(Brake)  "Brake"

== system CruiseControl/Subsystem2/Subsystem/rpm > 속도 ==
  회전수 [rpm] : Inport
  타이어 반경 : Inport  Port=2
  Data Type Conversion1 : DataTypeConversion  SaturateOnIntegerOverflow=off  RndMeth=Floor
  Gain : Gain  Gain=2*pi
  km/min > km/h : Product
  m->km : Constant  Value=1000
  m/min > km/min : Product  Inputs=*/
  min->hour : Constant  Value=60
  거리 계산 : Product
  속도 [km/h] : Outport
  wires:
  회전수 [rpm]/1 -> 거리 계산/1
  Gain/1 -> 거리 계산/2
  km/min > km/h/1 -> Data Type Conversion1/1
  min->hour/1 -> km/min > km/h/2
  m->km/1 -> m/min > km/min/2
  거리 계산/1 -> m/min > km/min/1
  타이어 반경/1 -> Gain/1
  m/min > km/min/1 -> km/min > km/h/1
  Data Type Conversion1/1 -> 속도 [km/h]/1

== system CruiseControl/Subsystem2/Torque Converter/각가속도 > 각속도 ==
  각가속도 [rad/sec^2] : Inport
  각속도 계산 : Integrator
  각속도 [rad/sec] : Outport
  wires:
  각속도 계산/1 -> 각속도 [rad/sec]/1
  각가속도 [rad/sec^2]/1 -> 각속도 계산/1

== system CruiseControl/Subsystem2/Torque Converter/각속도 > rpm ==
  rad/sec : Inport
  Constant : Constant  Value=2*pi
  Divide : Product  Inputs=*/
  Gain : Gain  Gain=60
  rpm : Outport
  wires:
  Gain/1 -> rpm/1
  rad/sec/1 -> Divide/1
  Constant/1 -> Divide/2
  Divide/1 -> Gain/1

== system CruiseControl/Subsystem2/Torque Converter/토크 > 각가속도 ==
  I [kgm^2] : Inport
  T [Nm] : Inport  Port=2
  Divide : Product  Inputs=*/
  W : Outport
  wires:
  T [Nm]/1 -> Divide/1
  I [kgm^2]/1 -> Divide/2
  Divide/1 -> W/1

== system CruiseControl/Subsystem2/Torque Converter/회전수 > 토크 ==
  엔진 회전수 Ne [rpm] : Inport
  출력 회전수 Nout [rpm] : Inport  Port=2
  Constant : Constant
  Constant1 : Constant  Value=-1
  MinMax : MinMax  Function=max  Inputs=2
  Relational Operator : RelationalOperator  OutDataTypeStr=boolean  RndMeth=Simplest  InputSameDT=off
  Subsystem : Subsystem
  Subsystem1 : Subsystem
  Switch : Switch  Criteria=u2 > Threshold  SaturateOnIntegerOverflow=off  InputSameDT=off
  균형 토크 Tout1 [Nm] : Outport
  출력 토크 Tout2 [Nm] : Outport  Port=2
  속도비 e : Outport  Port=3
  wires:
  MinMax/1 -> Subsystem1/1(엔진 회전수 Ne [rpm])
  Subsystem1/1(균형 토크 Tout1 [Nm]) -> 균형 토크 Tout1 [Nm]/1
  Subsystem1/2(출력 토크 Tout2 [Nm]) -> 출력 토크 Tout2 [Nm]/1
  Relational Operator/1 -> Switch/2
  Constant1/1 -> Switch/3
  출력 회전수 Nout [rpm]/1 -> Relational Operator/2, Subsystem/2(출력 회전수 Nout [rpm]), MinMax/2
  Constant/1 -> Switch/1
  Switch/1 -> Subsystem1/3(부호)
  엔진 회전수 Ne [rpm]/1 -> Relational Operator/1, Subsystem/1(엔진 회전수 Ne [rpm]), MinMax/1
  Subsystem/1(속도비 e) -> 속도비 e/1, Subsystem1/2(속도비 e)

== system CruiseControl/Subsystem2/변속기/Eighth ==
  gear : Inport
  pedal : Inport  Port=2
  car_speed : Inport  Port=3
  1-D Lookup Table1 : Lookup_n-D  NumberOfTableDimensions=1  BreakpointsForDimension1=[0 10 15 20 35 45 55 65 85 95 100]  Table=[59 59 60 65 90 120 150 155 220 280 280]  InternalRulePriority=Speed  RndMeth=Simplest
  Constant1 : Constant
  Relational Operator : RelationalOperator  Operator=<=  OutDataTypeStr=boolean  RndMeth=Simplest  InputSameDT=off
  Subtract : Sum  Inputs=+-
  Switch1 : Switch  Criteria=u2 > Threshold  SaturateOnIntegerOverflow=off  InputSameDT=off
  new_gear : Outport
  wires:
  Switch1/1 -> new_gear/1
  Subtract/1 -> Switch1/1
  car_speed/1 -> Relational Operator/1
  pedal/1 -> 1-D Lookup Table1/1
  1-D Lookup Table1/1 -> Relational Operator/2
  Relational Operator/1 -> Switch1/2
  gear/1 -> Subtract/1, Switch1/3
  Constant1/1 -> Subtract/2

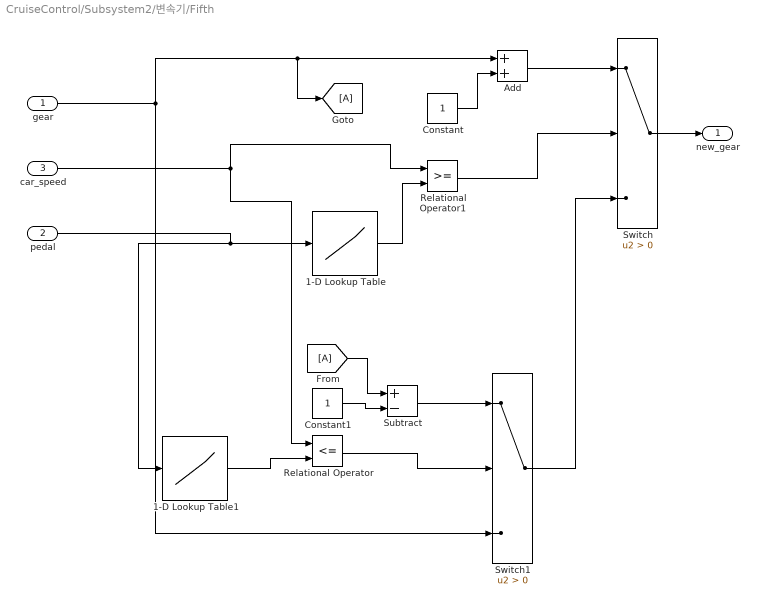
== system CruiseControl/Subsystem2/변속기/Fifth ==
  gear : Inport
  pedal : Inport  Port=2
  car_speed : Inport  Port=3
  1-D Lookup Table : Lookup_n-D  NumberOfTableDimensions=1  BreakpointsForDimension1=[0 4 8 20 25 30 45 75 85 95 100]  Table=[41 41 42 53 70 90 114 175 208 208 208]  InternalRulePriority=Speed  RndMeth=Simplest
  1-D Lookup Table1 : Lookup_n-D  NumberOfTableDimensions=1  BreakpointsForDimension1=[0 10 15 20 35 45 55 65 85 95 100]  Table=[24 24 25 28 30 35 50 68 135 166 166]  InternalRulePriority=Speed  RndMeth=Simplest
  Add : Sum
  Constant : Constant
  Constant1 : Constant
  From : From
  Goto : Goto
  Relational Operator : RelationalOperator  Operator=<=  OutDataTypeStr=boolean  RndMeth=Simplest  InputSameDT=off
  Relational Operator1 : RelationalOperator  OutDataTypeStr=boolean  RndMeth=Simplest  InputSameDT=off
  Subtract : Sum  Inputs=+-
  Switch : Switch  Criteria=u2 > Threshold  SaturateOnIntegerOverflow=off  InputSameDT=off
  Switch1 : Switch  Criteria=u2 > Threshold  SaturateOnIntegerOverflow=off  InputSameDT=off
  new_gear : Outport
  wires:
  Switch/1 -> new_gear/1
  Add/1 -> Switch/1
  Switch1/1 -> Switch/3
  Subtract/1 -> Switch1/1
  Relational Operator1/1 -> Switch/2
  car_speed/1 -> Relational Operator1/1, Relational Operator/1
  1-D Lookup Table/1 -> Relational Operator1/2
  pedal/1 -> 1-D Lookup Table1/1, 1-D Lookup Table/1
  1-D Lookup Table1/1 -> Relational Operator/2
  Relational Operator/1 -> Switch1/2
  gear/1 -> Goto/1, Add/1, Switch1/3
  Constant/1 -> Add/2
  From/1 -> Subtract/1
  Constant1/1 -> Subtract/2

== system CruiseControl/Subsystem2/변속기/First ==
  gear : Inport
  pedal : Inport  Port=2
  car_speed : Inport  Port=3
  Add : Sum
  Constant : Constant
  Relational Operator1 : RelationalOperator  OutDataTypeStr=boolean  RndMeth=Simplest  InputSameDT=off
  Switch : Switch  Criteria=u2 > Threshold  SaturateOnIntegerOverflow=off  InputSameDT=off
  shift12SP : Lookup_n-D  NumberOfTableDimensions=1  BreakpointsForDimension1=[0 4 8 20 25 30 45 75 85 95 100]  Table=[7 7 11 14 16 20 29 41 47 47 47]  InternalRulePriority=Speed  RndMeth=Simplest
  new_gear : Outport
  wires:
  Switch/1 -> new_gear/1
  Add/1 -> Switch/1
  Relational Operator1/1 -> Switch/2
  car_speed/1 -> Relational Operator1/1
  shift12SP/1 -> Relational Operator1/2
  pedal/1 -> shift12SP/1
  gear/1 -> [gear], Add/1
  Constant/1 -> Add/2
  [gear] -> Switch/3

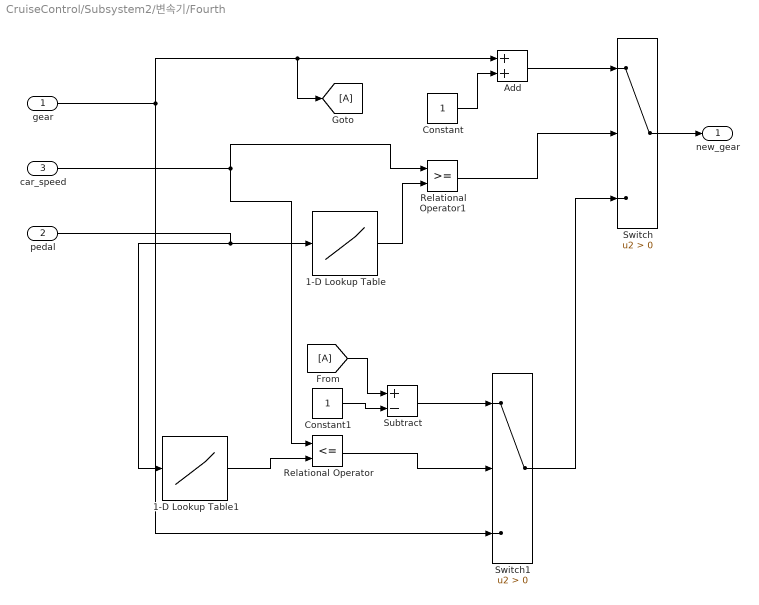
== system CruiseControl/Subsystem2/변속기/Fourth ==
  gear : Inport
  pedal : Inport  Port=2
  car_speed : Inport  Port=3
  1-D Lookup Table : Lookup_n-D  NumberOfTableDimensions=1  BreakpointsForDimension1=[0 4 8 20 25 30 45 75 85 95 100]  Table=[33 33 33 34 36 43 73 118 154 174 174]  InternalRulePriority=Speed  RndMeth=Simplest
  1-D Lookup Table1 : Lookup_n-D  NumberOfTableDimensions=1  BreakpointsForDimension1=[0 10 15 20 35 45 55 65 85 95 100]  Table=[14 14 20 20 20 30 40 50 80 122 122]  InternalRulePriority=Speed  RndMeth=Simplest
  Add : Sum
  Constant : Constant
  Constant1 : Constant
  From : From
  Goto : Goto
  Relational Operator : RelationalOperator  Operator=<=  OutDataTypeStr=boolean  RndMeth=Simplest  InputSameDT=off
  Relational Operator1 : RelationalOperator  OutDataTypeStr=boolean  RndMeth=Simplest  InputSameDT=off
  Subtract : Sum  Inputs=+-
  Switch : Switch  Criteria=u2 > Threshold  SaturateOnIntegerOverflow=off  InputSameDT=off
  Switch1 : Switch  Criteria=u2 > Threshold  SaturateOnIntegerOverflow=off  InputSameDT=off
  new_gear : Outport
  wires:
  Switch/1 -> new_gear/1
  Add/1 -> Switch/1
  Switch1/1 -> Switch/3
  Subtract/1 -> Switch1/1
  Relational Operator1/1 -> Switch/2
  car_speed/1 -> Relational Operator1/1, Relational Operator/1
  1-D Lookup Table/1 -> Relational Operator1/2
  pedal/1 -> 1-D Lookup Table1/1, 1-D Lookup Table/1
  1-D Lookup Table1/1 -> Relational Operator/2
  Relational Operator/1 -> Switch1/2
  gear/1 -> Goto/1, Add/1, Switch1/3
  Constant/1 -> Add/2
  From/1 -> Subtract/1
  Constant1/1 -> Subtract/2

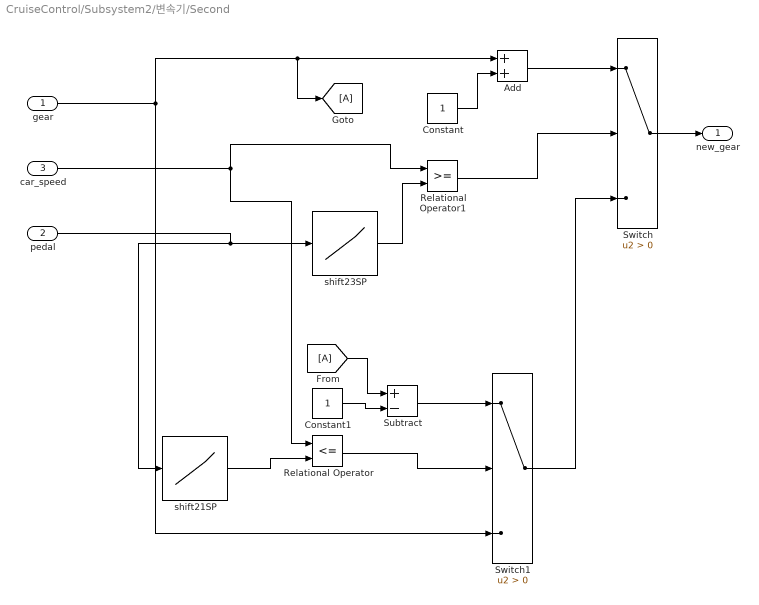
== system CruiseControl/Subsystem2/변속기/Second ==
  gear : Inport
  pedal : Inport  Port=2
  car_speed : Inport  Port=3
  Add : Sum
  Constant : Constant
  Constant1 : Constant
  From : From
  Goto : Goto
  Relational Operator : RelationalOperator  Operator=<=  OutDataTypeStr=boolean  RndMeth=Simplest  InputSameDT=off
  Relational Operator1 : RelationalOperator  OutDataTypeStr=boolean  RndMeth=Simplest  InputSameDT=off
  Subtract : Sum  Inputs=+-
  Switch : Switch  Criteria=u2 > Threshold  SaturateOnIntegerOverflow=off  InputSameDT=off
  Switch1 : Switch  Criteria=u2 > Threshold  SaturateOnIntegerOverflow=off  InputSameDT=off
  shift21SP : Lookup_n-D  NumberOfTableDimensions=1  BreakpointsForDimension1=[0 10 15 20 35 45 55 65 85 95 100]  Table=[5 5 5 5 5 5 5 5 20 25 30]  InternalRulePriority=Speed  RndMeth=Simplest
  shift23SP : Lookup_n-D  NumberOfTableDimensions=1  BreakpointsForDimension1=[0 4 8 20 25 30 45 75 85 95 100]  Table=[12 12 16 19 23 29 38 60 77 87 87]  InternalRulePriority=Speed  RndMeth=Simplest
  new_gear : Outport
  wires:
  Switch/1 -> new_gear/1
  Add/1 -> Switch/1
  Switch1/1 -> Switch/3
  Subtract/1 -> Switch1/1
  Relational Operator1/1 -> Switch/2
  car_speed/1 -> Relational Operator1/1, Relational Operator/1
  shift23SP/1 -> Relational Operator1/2
  pedal/1 -> shift21SP/1, shift23SP/1
  shift21SP/1 -> Relational Operator/2
  Relational Operator/1 -> Switch1/2
  gear/1 -> Goto/1, Add/1, Switch1/3
  Constant/1 -> Add/2
  From/1 -> Subtract/1
  Constant1/1 -> Subtract/2

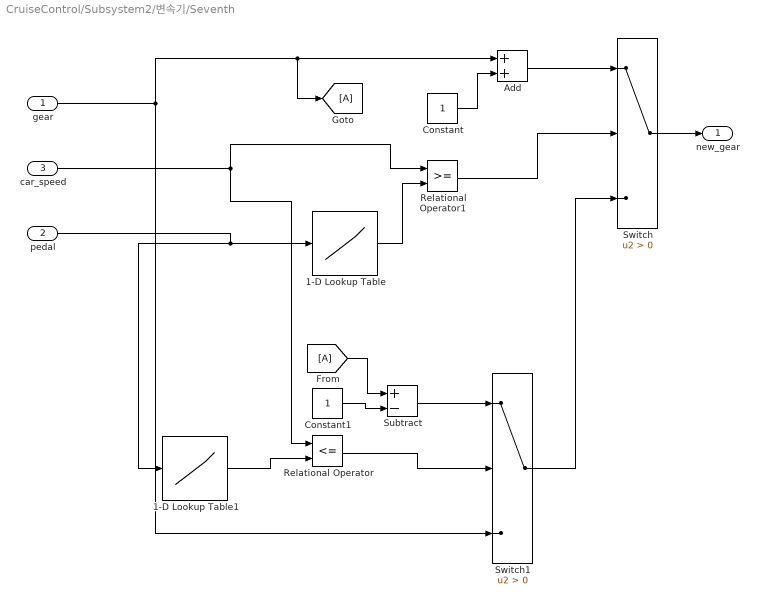
== system CruiseControl/Subsystem2/변속기/Seventh ==
  gear : Inport
  pedal : Inport  Port=2
  car_speed : Inport  Port=3
  1-D Lookup Table : Lookup_n-D  NumberOfTableDimensions=1  BreakpointsForDimension1=[0 4 8 20 25 30 45 75 85 95 100]  Table=[65 65 65 75 110 142 186 223 310 310 310]  InternalRulePriority=Speed  RndMeth=Simplest
  1-D Lookup Table1 : Lookup_n-D  NumberOfTableDimensions=1  BreakpointsForDimension1=[0 10 15 20 35 45 55 65 85 95 100]  Table=[43 43 43 43 60 70 80 135 211 225 225]  InternalRulePriority=Speed  RndMeth=Simplest
  Add : Sum
  Constant : Constant
  Constant1 : Constant
  From : From
  Goto : Goto
  Relational Operator : RelationalOperator  Operator=<=  OutDataTypeStr=boolean  RndMeth=Simplest  InputSameDT=off
  Relational Operator1 : RelationalOperator  OutDataTypeStr=boolean  RndMeth=Simplest  InputSameDT=off
  Subtract : Sum  Inputs=+-
  Switch : Switch  Criteria=u2 > Threshold  SaturateOnIntegerOverflow=off  InputSameDT=off
  Switch1 : Switch  Criteria=u2 > Threshold  SaturateOnIntegerOverflow=off  InputSameDT=off
  new_gear : Outport
  wires:
  Switch/1 -> new_gear/1
  Add/1 -> Switch/1
  Switch1/1 -> Switch/3
  Subtract/1 -> Switch1/1
  Relational Operator1/1 -> Switch/2
  car_speed/1 -> Relational Operator1/1, Relational Operator/1
  1-D Lookup Table/1 -> Relational Operator1/2
  pedal/1 -> 1-D Lookup Table1/1, 1-D Lookup Table/1
  1-D Lookup Table1/1 -> Relational Operator/2
  Relational Operator/1 -> Switch1/2
  gear/1 -> Goto/1, Add/1, Switch1/3
  Constant/1 -> Add/2
  From/1 -> Subtract/1
  Constant1/1 -> Subtract/2

== system CruiseControl/Subsystem2/변속기/Seventh1 ==
  gear : Inport
  pedal : Inport  Port=2
  car_speed : Inport  Port=3
  1-D Lookup Table : Lookup_n-D  NumberOfTableDimensions=1  BreakpointsForDimension1=[0 4 8 20 25 30 45 75 85 95 100]  Table=[49 49 55 65 85 115 150 200 235 255 255]  InternalRulePriority=Speed  RndMeth=Simplest
  1-D Lookup Table1 : Lookup_n-D  NumberOfTableDimensions=1  BreakpointsForDimension1=[0 10 15 20 35 45 55 65 85 95 100]  Table=[34 34 36 40 50 60 70 80 178 199 199]  InternalRulePriority=Speed  RndMeth=Simplest
  Add : Sum
  Constant : Constant
  Constant1 : Constant
  From : From
  Goto : Goto
  Relational Operator : RelationalOperator  Operator=<=  OutDataTypeStr=boolean  RndMeth=Simplest  InputSameDT=off
  Relational Operator1 : RelationalOperator  OutDataTypeStr=boolean  RndMeth=Simplest  InputSameDT=off
  Subtract : Sum  Inputs=+-
  Switch : Switch  Criteria=u2 > Threshold  SaturateOnIntegerOverflow=off  InputSameDT=off
  Switch1 : Switch  Criteria=u2 > Threshold  SaturateOnIntegerOverflow=off  InputSameDT=off
  new_gear : Outport
  wires:
  Switch/1 -> new_gear/1
  Add/1 -> Switch/1
  Switch1/1 -> Switch/3
  Subtract/1 -> Switch1/1
  Relational Operator1/1 -> Switch/2
  car_speed/1 -> Relational Operator1/1, Relational Operator/1
  1-D Lookup Table/1 -> Relational Operator1/2
  pedal/1 -> 1-D Lookup Table1/1, 1-D Lookup Table/1
  1-D Lookup Table1/1 -> Relational Operator/2
  Relational Operator/1 -> Switch1/2
  gear/1 -> Goto/1, Add/1, Switch1/3
  Constant/1 -> Add/2
  From/1 -> Subtract/1
  Constant1/1 -> Subtract/2

== system CruiseControl/Subsystem2/변속기/Third ==
  gear : Inport
  pedal : Inport  Port=2
  car_speed : Inport  Port=3
  1-D Lookup Table : Lookup_n-D  NumberOfTableDimensions=1  BreakpointsForDimension1=[0 4 8 20 25 30 45 75 85 95 100]  Table=[18 18 24 27 29 38 56 89 114 134 134]  InternalRulePriority=Speed  RndMeth=Simplest
  1-D Lookup Table1 : Lookup_n-D  NumberOfTableDimensions=1  BreakpointsForDimension1=[0 10 15 20 35 45 55 65 85 95 100]  Table=[10 10 10 10 10 10 10 25 35 50 75]  InternalRulePriority=Speed  RndMeth=Simplest
  Add : Sum
  Constant : Constant
  Constant1 : Constant
  From : From
  Goto : Goto
  Relational Operator : RelationalOperator  Operator=<=  OutDataTypeStr=boolean  RndMeth=Simplest  InputSameDT=off
  Relational Operator1 : RelationalOperator  OutDataTypeStr=boolean  RndMeth=Simplest  InputSameDT=off
  Subtract : Sum  Inputs=+-
  Switch : Switch  Criteria=u2 > Threshold  SaturateOnIntegerOverflow=off  InputSameDT=off
  Switch1 : Switch  Criteria=u2 > Threshold  SaturateOnIntegerOverflow=off  InputSameDT=off
  new_gear : Outport
  wires:
  Switch/1 -> new_gear/1
  Add/1 -> Switch/1
  Switch1/1 -> Switch/3
  Subtract/1 -> Switch1/1
  Relational Operator1/1 -> Switch/2
  car_speed/1 -> Relational Operator1/1, Relational Operator/1
  1-D Lookup Table/1 -> Relational Operator1/2
  pedal/1 -> 1-D Lookup Table1/1, 1-D Lookup Table/1
  1-D Lookup Table1/1 -> Relational Operator/2
  Relational Operator/1 -> Switch1/2
  gear/1 -> Goto/1, Add/1, Switch1/3
  Constant/1 -> Add/2
  From/1 -> Subtract/1
  Constant1/1 -> Subtract/2

== system CruiseControl/Subsystem/CC SPEED Calculator/CC_ON/A 동작 ==
  Current_CC_Speed : Inport
  Enable : EnablePort
  Add : Sum
  Constant : Constant  Value=2
  Saturation : Saturate  UpperLimit=110  LowerLimit=55
  Out1 : Outport
  wires:
  Current_CC_Speed/1 -> Add/1
  Constant/1 -> Add/2
  Add/1 -> Saturation/1
  Saturation/1 -> Out1/1

== system CruiseControl/Subsystem/CC SPEED Calculator/CC_ON/A,B 둘다동작X ==
  Current_CC_Speed : Inport
  Enable : EnablePort
  Out1 : Outport
  wires:
  Current_CC_Speed/1 -> Out1/1

== system CruiseControl/Subsystem/CC SPEED Calculator/CC_ON/B 동작 ==
  Current_CC_Speed : Inport
  Enable : EnablePort
  Add : Sum  Inputs=+-
  Constant : Constant  Value=2
  Saturation : Saturate  UpperLimit=110  LowerLimit=55
  Out1 : Outport
  wires:
  Constant/1 -> Add/2
  Current_CC_Speed/1 -> Add/1
  Add/1 -> Saturation/1
  Saturation/1 -> Out1/1

== system CruiseControl/Subsystem2/Subsystem/Subsystem2/Subsystem ==
  차량 속도 [km/h] : Inport
  Gain : Gain  Gain=1/2
  Product : Product
  Product1 : Product  Inputs=5
  km/h > m/s : Constant  Value=1000/3600
  공기 밀도 : Subsystem
  공기저항계수 : Constant  Value=0.35
  전면 투영 면적 [m^2] : Constant  Value=2.8
  주행저항 R [N] : Outport
  wires:
  공기 밀도/1(Out1) -> Product1/5
  Product1/1 -> Gain/1
  Gain/1 -> 주행저항 R [N]/1
  공기저항계수/1 -> Product1/3
  km/h > m/s/1 -> Product/2
  전면 투영 면적 [m^2]/1 -> Product1/4
  차량 속도 [km/h]/1 -> Product/1
  Product/1 -> Product1/2, Product1/1

== system CruiseControl/Subsystem2/Subsystem/Subsystem2/Subsystem1 ==
  경사 : Inport
  차량 중량 : Inport  Port=2
  Constant : Constant  Value=9.81
  Product : Product
  Product1 : Product
  Trigonometric Function : Trigonometry
  경사 저항 [N] : Outport
  wires:
  경사/1 -> Trigonometric Function/1
  Trigonometric Function/1 -> Product/1
  Product/1 -> Product1/1
  Product1/1 -> 경사 저항 [N]/1
  Constant/1 -> Product/2
  차량 중량/1 -> Product1/2

== system CruiseControl/Subsystem2/Subsystem/Subsystem2/Subsystem2 ==
  경사 : Inport
  차량 중량 : Inport  Port=2
  Constant : Constant  Value=9.81
  Product : Product  Inputs=4
  Trigonometric Function : Trigonometry  Operator=cos
  마찰 계수 : Constant  Value=0.01
  도로 저항 [N] : Outport
  wires:
  Constant/1 -> Product/2
  Trigonometric Function/1 -> Product/1
  경사/1 -> Trigonometric Function/1
  Product/1 -> 도로 저항 [N]/1
  차량 중량/1 -> Product/3
  마찰 계수/1 -> Product/4

== system CruiseControl/Subsystem2/Subsystem/Subsystem3/Subsystem1 ==
  토크 : Inport
  주행 저항 : Inport  Port=2
  타이어 반경 : Inport  Port=3
  Brake : Inport  Port=4
  Product : Product
  Subtract : Sum  Inputs=+-
  Subtract1 : Sum  Inputs=+-
  손실 포함 입력 토크 : Outport
  wires:
  토크/1 -> Subtract/1
  주행 저항/1 -> Product/1
  타이어 반경/1 -> Product/2
  Product/1 -> Subtract/2
  Subtract/1 -> Subtract1/1
  Brake/1 -> Subtract1/2
  Subtract1/1 -> 손실 포함 입력 토크/1

== system CruiseControl/Subsystem2/Subsystem/Subsystem3/각가속도 > 각속도 ==
  각가속도 [rad/sec^2] : Inport
  각속도 계산 : Integrator
  각속도 [rad/sec] : Outport
  wires:
  각속도 계산/1 -> 각속도 [rad/sec]/1
  각가속도 [rad/sec^2]/1 -> 각속도 계산/1

== system CruiseControl/Subsystem2/Subsystem/Subsystem3/각속도 > rpm ==
  rad/sec : Inport
  Constant : Constant  Value=2*pi
  Divide : Product  Inputs=*/
  Gain : Gain  Gain=60
  rpm : Outport
  wires:
  Divide/1 -> Gain/1
  Constant/1 -> Divide/2
  rad/sec/1 -> Divide/1
  Gain/1 -> rpm/1

== system CruiseControl/Subsystem2/Subsystem/Subsystem3/관성 계산 ==
  차량 중량 : Inport
  타이어 반경 : Inport  Port=2
  Product : Product
  Square : Math  Operator=square
  관성 : Outport
  wires:
  타이어 반경/1 -> Square/1
  차량 중량/1 -> Product/1
  Square/1 -> Product/2
  Product/1 -> 관성/1

== system CruiseControl/Subsystem2/Subsystem/Subsystem3/토크 > 각가속도 ==
  T [Nm] : Inport
  I [kgm^2] : Inport  Port=2
  Divide : Product  Inputs=*/
  W : Outport
  wires:
  T [Nm]/1 -> Divide/1
  I [kgm^2]/1 -> Divide/2
  Divide/1 -> W/1

== system CruiseControl/Subsystem2/Torque Converter/회전수 > 토크/Subsystem ==
  엔진 회전수 Ne [rpm] : Inport
  출력 회전수 Nout [rpm] : Inport  Port=2
  Compare To Zero2 : simulink/Logic and Bit Operations/Compare To Zero  relop===  OutDataTypeStr=boolean
  Compare To Zero3 : simulink/Logic and Bit Operations/Compare To Zero  relop===  OutDataTypeStr=boolean
  Constant1 : Constant  Value=0
  Divide2 : Product  Inputs=*/
  Divide3 : Product  Inputs=*/
  From1 : From
  Goto1 : Goto
  Logical Operator : Logic  Operator=OR  AllPortsSameDT=off  OutDataTypeStr=boolean
  MinMax1 : MinMax  Inputs=2
  Saturation3 : Saturate  UpperLimit=10000  LowerLimit=1
  Saturation4 : Saturate  UpperLimit=10000  LowerLimit=1
  Saturation5 : Saturate  UpperLimit=1  LowerLimit=0
  Switch1 : Switch  Criteria=u2 > Threshold  SaturateOnIntegerOverflow=off  InputSameDT=off
  속도비 e : Outport
  wires:
  Divide3/1 -> MinMax1/2
  Switch1/1 -> 속도비 e/1
  MinMax1/1 -> Saturation5/1
  Logical Operator/1 -> Switch1/2
  Saturation5/1 -> Switch1/3
  From1/1 -> Divide2/1
  Compare To Zero3/1 -> Logical Operator/2
  Saturation4/1 -> Goto1/1, Divide3/2
  Compare To Zero2/1 -> Logical Operator/1
  Saturation3/1 -> Divide3/1, Divide2/2
  Constant1/1 -> Switch1/1
  Divide2/1 -> MinMax1/1
  엔진 회전수 Ne [rpm]/1 -> Saturation3/1, Compare To Zero2/1
  출력 회전수 Nout [rpm]/1 -> Saturation4/1, Compare To Zero3/1

== system CruiseControl/Subsystem2/Torque Converter/회전수 > 토크/Subsystem1 ==
  엔진 회전수 Ne [rpm] : Inport
  속도비 e : Inport  Port=2
  부호 : Inport  Port=3
  Math Function : Math  Operator=magnitude^2
  Product : Product
  Product1 : Product
  Product2 : Product
  TratioMap : Lookup_n-D  NumberOfTableDimensions=1  BreakpointsForDimension1=[0;0.1;0.2;0.3;0.4;0.5;0.6;0.7;0.8;0.85;0.9;0.95;0.98;1]  Table=[2.240 2.100 1.970 1.835 1.685 1.530 1.370 1.220 1.085 1.005 1.000 1.000 0.997 1.000]  InternalRulePriority=Speed  RndMeth=Simplest
  capacityMap : Lookup_n-D  NumberOfTableDimensions=1  BreakpointsForDimension1=[0;0.1;0.2;0.3;0.4;0.5;0.6;0.7;0.8;0.85;0.9;0.95;0.98;1]  Table=[2.835e-05 2.81e-05 2.704e-05 2.607e-05 2.508e-05 2.383e-05 2.226e-05 2.135e-05 1.881e-05 1.741e-05 1.245e-05 6.5e-06 2.6e-06 0]  InternalRulePriority=Speed  RndMeth=Simplest
  균형 토크 Tout1 [Nm] : Outport
  출력 토크 Tout2 [Nm] : Outport  Port=2
  wires:
  엔진 회전수 Ne [rpm]/1 -> Math Function/1
  속도비 e/1 -> TratioMap/1, capacityMap/1
  Math Function/1 -> Product/1
  capacityMap/1 -> Product/2
  Product/1 -> Product1/1
  부호/1 -> Product1/2
  Product1/1 -> Product2/1, 균형 토크 Tout1 [Nm]/1
  TratioMap/1 -> Product2/2
  Product2/1 -> 출력 토크 Tout2 [Nm]/1

== system CruiseControl/Subsystem2/Subsystem/Subsystem2/Subsystem/공기 밀도 ==
  Add : Sum
  Constant : Constant  Value=1.293
  Constant1 : Constant  Value=273.15
  Constant2 : Constant  Value=25
  Constant3 : Constant  Value=1013.25
  Constant4 : Constant  Value=1013.25
  Divide : Product  Inputs=*/
  Divide1 : Product  Inputs=*/
  Product1 : Product  Inputs=3
  Out1 : Outport
  wires:
  Divide/1 -> Product1/2
  Constant4/1 -> Divide1/2
  Constant3/1 -> Divide1/1
  Constant1/1 -> Add/1, Divide/1
  Constant2/1 -> Add/2
  Add/1 -> Divide/2
  Divide1/1 -> Product1/3
  Constant/1 -> Product1/1
  Product1/1 -> Out1/1
